simulink model "chinmay_sir"  (R2023a)
settings: Solver=VariableStepAuto  StartTime=0.0  StopTime=10.0  RelTol=1e-3
libraries: roblocks x2
settings Model: Creator=Tech Land  LastModifiedBy=Tech Land

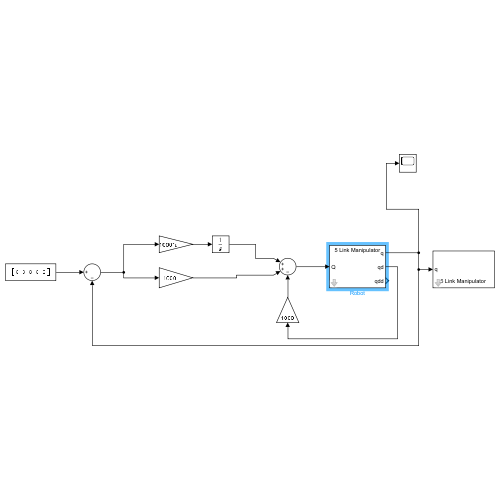
[thumbnail: Simulink's stored preview of the top-level diagram]
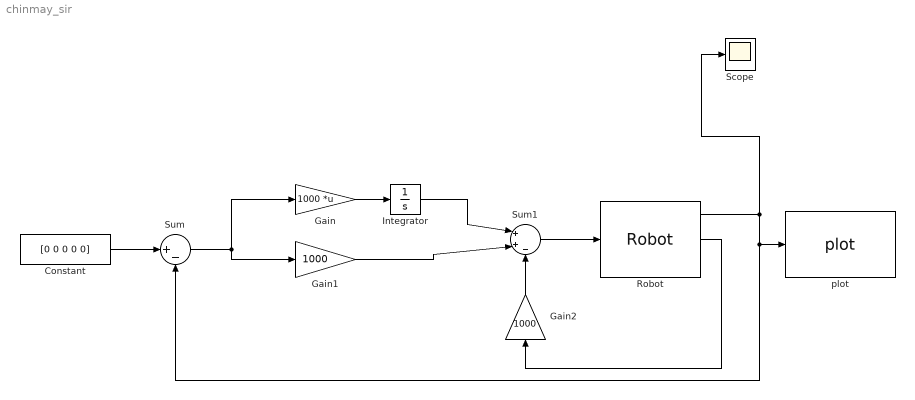
== system chinmay_sir ==
  Constant : Constant  Value=[0 0 0 0 0]
  Gain : Gain  Gain=1000  Multiplication=Matrix(K*u)
  Gain1 : Gain  Gain=1000
  Gain2 : Gain  Gain=1000
  Integrator : Integrator
  Robot : roblocks/Arm/Robot  robot=robot  q0=[0 0 0 0 0]
      link override S-Function: FunctionName=slaccel
  Scope : Scope
  Sum : Sum  Inputs=|+-
  Sum1 : Sum  Inputs=|++-
  plot : roblocks/Arm/plot  robot=robot  fps=60  holdplot=on
  wires:
  Gain1/1 -> Sum1/2
  Robot/1 -> Scope/1, plot/1, Sum/2
  Sum/1 -> Gain/1, Gain1/1
  Constant/1 -> Sum/1
  Gain/1 -> Integrator/1
  Integrator/1 -> Sum1/1
  Robot/2 -> Gain2/1
  Gain2/1 -> Sum1/3
  Sum1/1 -> Robot/1
